simulink model "IM_RotateCircuit"  (R2019b)
settings: Solver=VariableStepAuto  StartTime=0.0  StopTime=100  RelTol=1e-3
InitFcn:
  | run('MotorParamInit.m');
values from neighbouring files (symbols this model uses):
  Llr = Lls    (= 0.06396484375)    [MotorParamInit.m]
  Lls = 262/4096    (= 0.06396484375)    [MotorParamInit.m]
  Lm = 5793/4096    (= 1.41430664062)    [MotorParamInit.m]
  Lr = Lm+Llr    (= 1.47827148438)    [MotorParamInit.m]
  Ls = Lm+Lls    (= 1.47827148438)    [MotorParamInit.m]
  Rr = 81/4096    (= 0.019775390625)    [MotorParamInit.m]
  Rs = 100/4096    (= 0.0244140625)    [MotorParamInit.m]
  Vsd = 0.1    [MotorParamInit.m]
  Ws = 0.1    [MotorParamInit.m]
libraries: powerlib x30
settings Model: Creator=W002220B  LastModifiedBy=W002220B
settings SolverCC: AlgebraicLoopSolver=LineSearch

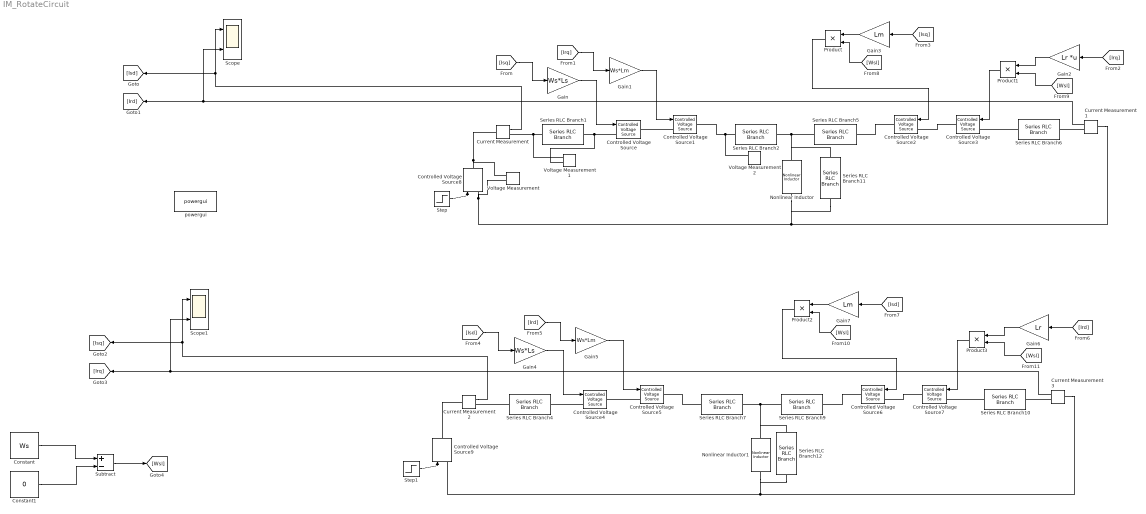
== system IM_RotateCircuit ==
  Constant : Constant  Value=Ws
  Constant1 : Constant  Value=0
  Controlled Voltage Source{,1..9} (10 alike) : powerlib/Electrical Sources/Controlled Voltage Source  Initialize=on  Source_Type=DC  Amplitude=0  Phase=0  Frequency=0  Measurements=None
      settings: SourceProductName=Simscape Electrical
  Current Measurement{,1..3} (4 alike) : powerlib/Measurements/Current Measurement  PhasorSimulation=off  OutputType=Complex  PSBequivalent=0
      settings: SourceProductName=Simscape Electrical
  Gain : Gain  Gain=Ws*Ls
  Gain1 : Gain  Gain=Ws*Lm
  Gain2 : Gain  Gain=Lr  Multiplication=Matrix(K*u)
  Gain3 : Gain  Gain=Lm
  Gain4 : Gain  Gain=Ws*Ls
  Gain5 : Gain  Gain=Ws*Lm
  Gain6 : Gain  Gain=Lr
  Gain7 : Gain  Gain=Lm
  Nonlinear Inductor : powerlib/Elements/Nonlinear Inductor  DiscreteSolver=Backward Euler  VI=MagCurve  IFL=0  Measurements=None
      settings: SourceProductName=Simscape Electrical  SourceProductBaseCode=PS
  Nonlinear Inductor1 : powerlib/Elements/Nonlinear Inductor  DiscreteSolver=Backward Euler  VI=MagCurve  IFL=0  Measurements=None
      settings: SourceProductName=Simscape Electrical  SourceProductBaseCode=PS
  Product{,1..3} (4 alike) : Product
  Scope : Scope  NumInputPorts=2
  Scope1 : Scope  NumInputPorts=2
  Series RLC Branch1 : powerlib/Elements/Series RLC Branch  LConnTagsString=__new0  RConnTagsString=__new0  BranchType=R  Resistance=Rs  Inductance=1e-3  SetiL0=off  InitialCurrent=0  Capacitance=1e-6  Setx0=off  InitialVoltage=0  Measurements=None
      settings: SourceProductName=Simscape Electrical
  Series RLC Branch10 : powerlib/Elements/Series RLC Branch  LConnTagsString=__new0  RConnTagsString=__new0  BranchType=R  Resistance=Rr  Inductance=1e-3  SetiL0=off  InitialCurrent=0  Capacitance=1e-6  Setx0=off  InitialVoltage=0  Measurements=None
      settings: SourceProductName=Simscape Electrical
  Series RLC Branch11 : powerlib/Elements/Series RLC Branch  LConnTagsString=__new0  RConnTagsString=__new0  BranchType=R  Resistance=10000  Inductance=Lm  SetiL0=off  InitialCurrent=0  Capacitance=1e-6  Setx0=off  InitialVoltage=0  Measurements=None
      settings: SourceProductName=Simscape Electrical
  Series RLC Branch12 : powerlib/Elements/Series RLC Branch  LConnTagsString=__new0  RConnTagsString=__new0  BranchType=R  Resistance=10000  Inductance=Lm  SetiL0=off  InitialCurrent=0  Capacitance=1e-6  Setx0=off  InitialVoltage=0  Measurements=None
      settings: SourceProductName=Simscape Electrical
  Series RLC Branch2 : powerlib/Elements/Series RLC Branch  LConnTagsString=__new0  RConnTagsString=__new0  BranchType=L  Resistance=1  Inductance=Lls  SetiL0=off  InitialCurrent=0  Capacitance=1e-6  Setx0=off  InitialVoltage=0  Measurements=None
      settings: SourceProductName=Simscape Electrical
  Series RLC Branch4 : powerlib/Elements/Series RLC Branch  LConnTagsString=__new0  RConnTagsString=__new0  BranchType=R  Resistance=Rs  Inductance=1e-3  SetiL0=off  InitialCurrent=0  Capacitance=1e-6  Setx0=off  InitialVoltage=0  Measurements=None
      settings: SourceProductName=Simscape Electrical
  Series RLC Branch5 : powerlib/Elements/Series RLC Branch  LConnTagsString=__new0  RConnTagsString=__new0  BranchType=L  Resistance=1  Inductance=Llr  SetiL0=off  InitialCurrent=0  Capacitance=1e-6  Setx0=off  InitialVoltage=0  Measurements=None
      settings: SourceProductName=Simscape Electrical
  Series RLC Branch6 : powerlib/Elements/Series RLC Branch  LConnTagsString=__new0  RConnTagsString=__new0  BranchType=R  Resistance=Rr  Inductance=1e-3  SetiL0=off  InitialCurrent=0  Capacitance=1e-6  Setx0=off  InitialVoltage=0  Measurements=None
      settings: SourceProductName=Simscape Electrical
  Series RLC Branch7 : powerlib/Elements/Series RLC Branch  LConnTagsString=__new0  RConnTagsString=__new0  BranchType=L  Resistance=1  Inductance=Lls  SetiL0=off  InitialCurrent=0  Capacitance=1e-6  Setx0=off  InitialVoltage=0  Measurements=None
      settings: SourceProductName=Simscape Electrical
  Series RLC Branch9 : powerlib/Elements/Series RLC Branch  LConnTagsString=__new0  RConnTagsString=__new0  BranchType=L  Resistance=1  Inductance=Llr  SetiL0=off  InitialCurrent=0  Capacitance=1e-6  Setx0=off  InitialVoltage=0  Measurements=None
      settings: SourceProductName=Simscape Electrical
  Step : Step  Time=0.1  After=Vsd  SampleTime=0
  Step1 : Step  Time=0.1  After=Vsd  SampleTime=0
  Subtract : Sum  Inputs=+-
  Voltage Measurement : powerlib/Measurements/Voltage Measurement  PhasorSimulation=off  OutputType=Complex  PSBequivalent=0
      settings: SourceProductName=Simscape Electrical
  Voltage Measurement1 : powerlib/Measurements/Voltage Measurement  PhasorSimulation=off  OutputType=Complex  PSBequivalent=0
      settings: SourceProductName=Simscape Electrical
  Voltage Measurement2 : powerlib/Measurements/Voltage Measurement  PhasorSimulation=off  OutputType=Complex  PSBequivalent=0
      settings: SourceProductName=Simscape Electrical
  powergui : powerlib/powergui  Priority=1  SimulationMode=Discrete  SampleTime=500e-6  frequency=60  Iterations=50  frequencyindice=0  Pbase=100e6  ErrMax=1e-4  UnitsV=kV  UnitsW=MW  buscounter=0  FunctionMessages=off  echomessages=off  EnableUseOfTLC=off  CurrentSourceSwitches=off  DisableSnubberDevices=off  DisableRonSwitches=off  DisableVfSwitches=off  DisplayEquations=off  AutomaticDiscreteSolvers=off  SolverType=Tustin/Backward Euler (TBE)  Interpol=off  ExternalGateDelay=off  methode=off  Ts=100  x0status=blocks  SPID=on  SwTol=0  HookPort=off  NonlinearTolerance=1e-4  nMaxIteration=100  ContinueOnMaxIteration=off  RestoreLinks=warning  ResistiveCurrentMeasurement=off  Frange=[0:2:500]  Ylog=off  Xlog=on  ShowGrid=off  save=off  variable=ZData  structure=0  ZoomFFT=off  StartTime=0.0  cycles=1  DisplayStyle=1  fundamental=60  FreqAxis=off  MaxFrequency=1000  frequencyindicesteady=1  RmsSteady=1  display=off
      settings: SourceProductName=Simscape Electrical
  wires:
  Current Measurement/1 -> [Isd], Scope/1
  Current Measurement1/1 -> [Ird], Scope/2
  [Isq] -> Gain/1
  [Irq] -> Gain1/1
  Gain/1 -> Controlled Voltage Source/1
  Gain1/1 -> Controlled Voltage Source1/1
  [Isq] -> Gain3/1
  Gain5/1 -> Controlled Voltage Source5/1
  Gain4/1 -> Controlled Voltage Source4/1
  [Ird] -> Gain5/1
  [Isd] -> Gain4/1
  Current Measurement3/1 -> Scope1/2, [Irq]
  Current Measurement2/1 -> Scope1/1, [Isq]
  Constant/1 -> Subtract/1
  Constant1/1 -> Subtract/2
  Subtract/1 -> [Wsl]
  Gain3/1 -> Product/1
  Product/1 -> Controlled Voltage Source2/1
  [Wsl] -> Product/2
  [Wsl] -> Product1/2
  Gain2/1 -> Product1/1
  [Irq] -> Gain2/1
  Product1/1 -> Controlled Voltage Source3/1
  Product3/1 -> Controlled Voltage Source7/1
  [Ird] -> Gain6/1
  Gain6/1 -> Product3/1
  [Wsl] -> Product3/2
  [Wsl] -> Product2/2
  Product2/1 -> Controlled Voltage Source6/1
  Gain7/1 -> Product2/1
  [Isd] -> Gain7/1
  Step/1 -> Controlled Voltage Source8/1
  Step1/1 -> Controlled Voltage Source9/1
  connections:
  Controlled Voltage Source8/RConn1 -- Current Measurement/LConn1 -- Voltage Measurement/LConn1
  Series RLC Branch1/LConn1 -- Voltage Measurement1/LConn1 -- Current Measurement/RConn1
  Controlled Voltage Source/LConn1 -- Voltage Measurement1/LConn2 -- Series RLC Branch1/RConn1
  Controlled Voltage Source1/LConn1 -- Controlled Voltage Source/RConn1
  Series RLC Branch2/LConn1 -- Voltage Measurement2/LConn1 -- Controlled Voltage Source1/RConn1
  Series RLC Branch5/LConn1 -- Series RLC Branch11/LConn1 -- Nonlinear Inductor/RConn1 -- Series RLC Branch2/RConn1
  Controlled Voltage Source2/RConn1 -- Series RLC Branch5/RConn1
  Controlled Voltage Source3/RConn1 -- Controlled Voltage Source2/LConn1
  Series RLC Branch6/LConn1 -- Controlled Voltage Source3/LConn1
  Current Measurement1/LConn1 -- Series RLC Branch11/RConn1 -- Nonlinear Inductor/LConn1 -- Voltage Measurement/LConn2 -- Controlled Voltage Source8/LConn1
  Current Measurement1/RConn1 -- Series RLC Branch6/RConn1
  Series RLC Branch9/LConn1 -- Series RLC Branch12/LConn1 -- Nonlinear Inductor1/RConn1 -- Series RLC Branch7/RConn1
  Current Measurement3/LConn1 -- Series RLC Branch12/RConn1 -- Nonlinear Inductor1/LConn1 -- Controlled Voltage Source9/LConn1
  Current Measurement3/RConn1 -- Series RLC Branch10/RConn1
  Controlled Voltage Source7/RConn1 -- Controlled Voltage Source6/LConn1
  Controlled Voltage Source5/LConn1 -- Controlled Voltage Source4/RConn1
  Controlled Voltage Source4/LConn1 -- Series RLC Branch4/RConn1
  Series RLC Branch4/LConn1 -- Current Measurement2/RConn1
  Series RLC Branch7/LConn1 -- Controlled Voltage Source5/RConn1
  Controlled Voltage Source6/RConn1 -- Series RLC Branch9/RConn1
  Controlled Voltage Source9/RConn1 -- Current Measurement2/LConn1
  Series RLC Branch10/LConn1 -- Controlled Voltage Source7/LConn1
